simulink model "AMR_MoboticControlUnit_23b"  (R2023b)
settings: Solver=VariableStepAuto  StartTime=0.0  StopTime=10.0  RelTol=1e-3
values from neighbouring files (symbols this model uses):
  vehicle_track = 877    [param.mat]
  vehicle_wheelbase = 2367    [param.mat]
undefined symbols (not defined in the file or in its folder): boost_speed_multiplier, max_speed_multiplier
libraries: simulink_extras x3
settings Model: Creator=matlab.cut  LastModifiedBy=matlab.cut

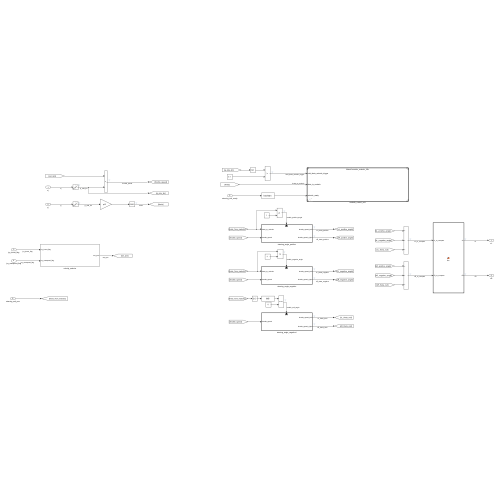
[thumbnail: Simulink's stored preview of the top-level diagram]
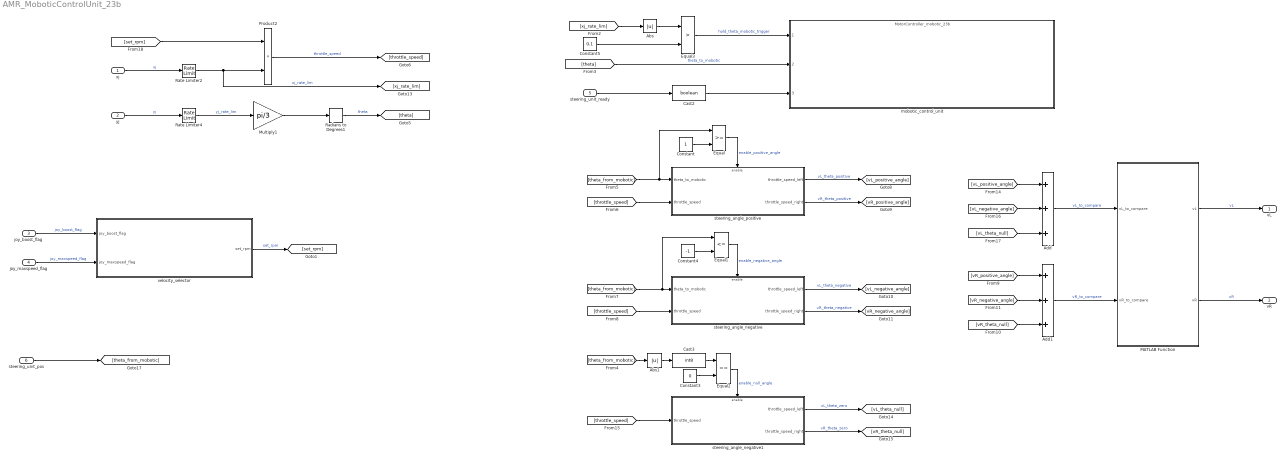
== system AMR_MoboticControlUnit_23b ==
  xj : Inport
  yj : Inport  Port=2
  joy_boost_flag : Inport  Port=3
  joy_maxspeed_flag : Inport  Port=4
  steering_unit_ready : Inport  Port=5
  steering_unit_pos : Inport  Port=6
  Abs : Abs  SaturateOnIntegerOverflow=off
  Abs1 : Abs  SaturateOnIntegerOverflow=off
  Add : Sum  Inputs=+++
  Add1 : Sum  Inputs=+++
  Cast2 : DataTypeConversion  OutDataTypeStr=boolean  SaturateOnIntegerOverflow=off  RndMeth=Floor
  Cast3 : DataTypeConversion  OutDataTypeStr=int8  SaturateOnIntegerOverflow=off  RndMeth=Floor
  Constant : Constant
  Constant3 : Constant  Value=0
  Constant4 : Constant  Value=-1
  Constant5 : Constant  Value=0.1
  Equal : RelationalOperator  OutDataTypeStr=boolean  RndMeth=Simplest  InputSameDT=off
  Equal1 : RelationalOperator  Operator=<=  OutDataTypeStr=boolean  RndMeth=Simplest  InputSameDT=off
  Equal2 : RelationalOperator  Operator===  OutDataTypeStr=boolean  RndMeth=Simplest  InputSameDT=off
  Equal3 : RelationalOperator  Operator=>  OutDataTypeStr=boolean  RndMeth=Simplest  InputSameDT=off
  MATLAB Function : MATLAB Function  TreatAsAtomicUnit=on
  Multiply1 : Gain  Gain=pi/3
  Product2 : Product
  Radians to Degrees1 : simulink_extras/Transformations/Radians to Degrees
  Rate Limiter2 : RateLimiter  SampleTimeMode=inherited
  Rate Limiter4 : RateLimiter  RisingSlewLimit=0.8  FallingSlewLimit=-0.8  SampleTimeMode=inherited
  mobotic_control_unit : ModelReference  ModelNameDialog=MotorController_mobotic_23b.slx  SimulationMode=Normal  ModelReferenceVersion=1.44
  steering_angle_negative : Subsystem
  steering_angle_negative1 : Subsystem
  steering_angle_positive : Subsystem
  velocity_selector : Subsystem
  vL : Outport
  vR : Outport  Port=2
  wires:
  [theta_from_mobotic] -> Abs1/1
  Abs1/1 -> Cast3/1
  steering_unit_ready/1 -> Cast2/1
  yj/1 -> Rate Limiter4/1  "yj"
  Cast2/1 -> mobotic_control_unit/3
  Rate Limiter2/1 -> [xj_rate_lim], Product2/2  "xj_rate_lim"
  [throttle_speed] -> steering_angle_negative1/1(throttle_speed)
  Abs/1 -> Equal3/1
  MATLAB Function/1(vL) -> vL/1  "vL"
  Add1/1 -> MATLAB Function/2(vR_to_compare)  "vR_to_compare"
  Constant4/1 -> Equal1/2
  Equal/1 -> steering_angle_positive/Enable  "enable_positive_angle"
  [vL_theta_null] -> Add/3
  steering_unit_pos/1 -> [theta_from_mobotic]
  [theta_from_mobotic] -> Equal/1, steering_angle_positive/1(theta_to_mobotic)
  Product2/1 -> [throttle_speed]  "throttle_speed"
  Constant3/1 -> Equal2/2
  [set_rpm] -> Product2/1
  [vL_negative_angle] -> Add/2
  Equal3/1 -> mobotic_control_unit/1  "hold_theta_mobotic_trigger"
  [vR_theta_null] -> Add1/3
  Cast3/1 -> Equal2/1
  [vR_negative_angle] -> Add1/2
  MATLAB Function/2(vR) -> vR/1  "vR"
  Rate Limiter4/1 -> Multiply1/1  "yj_rate_lim"
  steering_angle_negative/1(throttle_speed_left) -> [vL_negative_angle]  "vL_theta_negative"
  Constant/1 -> Equal/2
  xj/1 -> Rate Limiter2/1  "xj"
  [vR_positive_angle] -> Add1/1
  Constant5/1 -> Equal3/2
  steering_angle_positive/2(throttle_speed_right) -> [vR_positive_angle]  "vR_theta_positive"
  [xj_rate_lim] -> Abs/1
  [theta_from_mobotic] -> steering_angle_negative/1(theta_to_mobotic), Equal1/1
  steering_angle_negative/2(throttle_speed_right) -> [vR_negative_angle]  "vR_theta_negative"
  Radians to Degrees1/1 -> [theta]  "theta"
  Add/1 -> MATLAB Function/1(vL_to_compare)  "vL_to_compare"
  Equal2/1 -> steering_angle_negative1/Enable  "enable_null_angle"
  [vL_positive_angle] -> Add/1
  steering_angle_negative1/1(throttle_speed_left) -> [vL_theta_null]  "vL_theta_zero"
  [theta] -> mobotic_control_unit/2  "theta_to_mobotic"
  [throttle_speed] -> steering_angle_negative/2(throttle_speed)
  Multiply1/1 -> Radians to Degrees1/1
  steering_angle_positive/1(throttle_speed_left) -> [vL_positive_angle]  "vL_theta_positive"
  Equal1/1 -> steering_angle_negative/Enable  "enable_negative_angle"
  steering_angle_negative1/2(throttle_speed_right) -> [vR_theta_null]  "vR_theta_zero"
  [throttle_speed] -> steering_angle_positive/2(throttle_speed)
  velocity_selector/1(set_rpm) -> [set_rpm]  "set_rpm"
  joy_boost_flag/1 -> velocity_selector/1(joy_boost_flag)  "joy_boost_flag"
  joy_maxspeed_flag/1 -> velocity_selector/2(joy_maxspeed_flag)  "joy_maxspeed_flag"

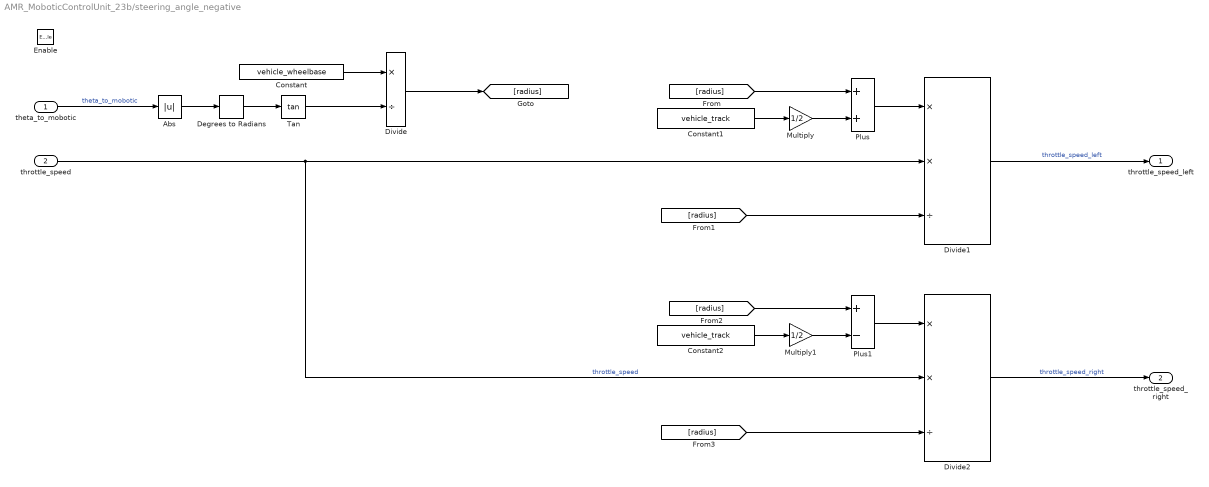
== system AMR_MoboticControlUnit_23b/steering_angle_negative ==
  theta_to_mobotic : Inport
  throttle_speed : Inport  Port=2
  Enable : EnablePort
  Abs : Abs  SaturateOnIntegerOverflow=off
  Constant : Constant  Value=vehicle_wheelbase
  Constant1 : Constant  Value=vehicle_track
  Constant2 : Constant  Value=vehicle_track
  Degrees to Radians : simulink_extras/Transformations/Degrees to Radians
  Divide : Product  Inputs=*/
  Divide1 : Product  Inputs=**/
  Divide2 : Product  Inputs=**/
  Multiply : Gain  Gain=1/2
  Multiply1 : Gain  Gain=1/2
  Plus : Sum
  Plus1 : Sum  Inputs=+-
  Tan : Trigonometry  Operator=tan
  throttle_speed_left : Outport  OutputWhenDisabled=reset  InitialOutput=[0]
  throttle_speed_right : Outport  Port=2  OutputWhenDisabled=reset  InitialOutput=[0]
  wires:
  Constant2/1 -> Multiply1/1
  Plus1/1 -> Divide2/1
  throttle_speed/1 -> Divide1/2, Divide2/2  "throttle_speed"
  Divide2/1 -> throttle_speed_right/1  "throttle_speed_right"
  [radius] -> Plus1/1
  Multiply1/1 -> Plus1/2
  [radius] -> Divide2/3
  [radius] -> Divide1/3
  Multiply/1 -> Plus/2
  [radius] -> Plus/1
  Divide1/1 -> throttle_speed_left/1  "throttle_speed_left"
  Plus/1 -> Divide1/1
  Constant1/1 -> Multiply/1
  Tan/1 -> Divide/2
  Divide/1 -> [radius]
  Constant/1 -> Divide/1
  Degrees to Radians/1 -> Tan/1
  Abs/1 -> Degrees to Radians/1
  theta_to_mobotic/1 -> Abs/1  "theta_to_mobotic"

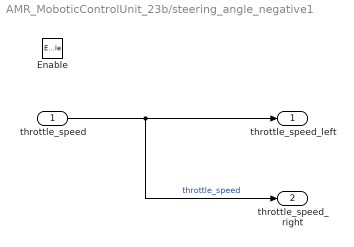
== system AMR_MoboticControlUnit_23b/steering_angle_negative1 ==
  throttle_speed : Inport
  Enable : EnablePort
  throttle_speed_left : Outport  OutputWhenDisabled=reset  InitialOutput=[0]
  throttle_speed_right : Outport  Port=2  OutputWhenDisabled=reset  InitialOutput=[0]
  wires:
  throttle_speed/1 -> throttle_speed_right/1, throttle_speed_left/1  "throttle_speed"

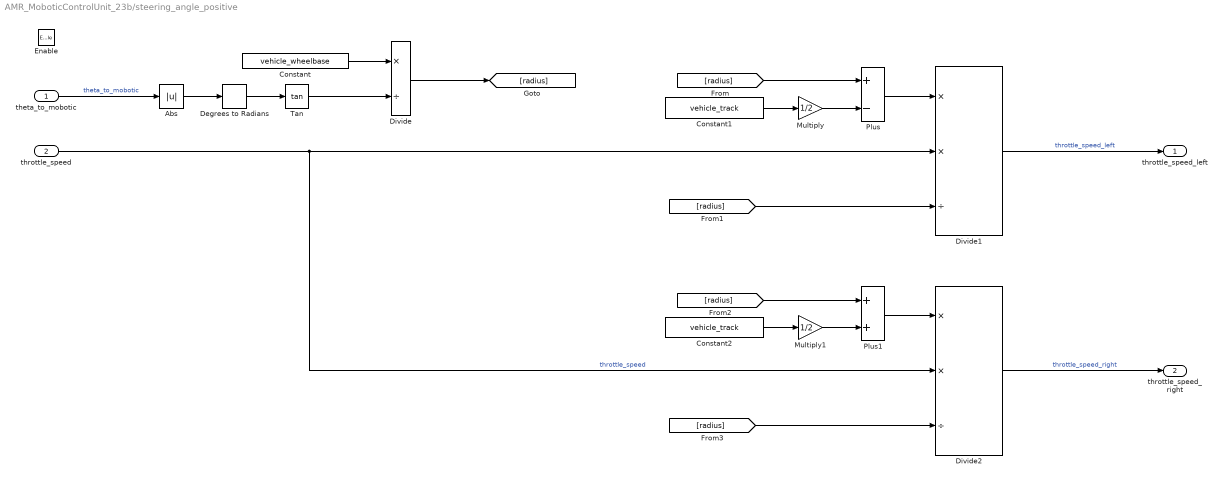
== system AMR_MoboticControlUnit_23b/steering_angle_positive ==
  theta_to_mobotic : Inport
  throttle_speed : Inport  Port=2
  Enable : EnablePort
  Abs : Abs  SaturateOnIntegerOverflow=off
  Constant : Constant  Value=vehicle_wheelbase
  Constant1 : Constant  Value=vehicle_track
  Constant2 : Constant  Value=vehicle_track
  Degrees to Radians : simulink_extras/Transformations/Degrees to Radians
  Divide : Product  Inputs=*/
  Divide1 : Product  Inputs=**/
  Divide2 : Product  Inputs=**/
  Multiply : Gain  Gain=1/2
  Multiply1 : Gain  Gain=1/2
  Plus : Sum  Inputs=+-
  Plus1 : Sum
  Tan : Trigonometry  Operator=tan
  throttle_speed_left : Outport  OutputWhenDisabled=reset  InitialOutput=[0]
  throttle_speed_right : Outport  Port=2  OutputWhenDisabled=reset  InitialOutput=[0]
  wires:
  theta_to_mobotic/1 -> Abs/1  "theta_to_mobotic"
  Abs/1 -> Degrees to Radians/1
  Degrees to Radians/1 -> Tan/1
  Constant/1 -> Divide/1
  Divide/1 -> [radius]
  Tan/1 -> Divide/2
  Constant1/1 -> Multiply/1
  Plus/1 -> Divide1/1
  Divide1/1 -> throttle_speed_left/1  "throttle_speed_left"
  [radius] -> Plus/1
  Multiply/1 -> Plus/2
  [radius] -> Divide1/3
  [radius] -> Divide2/3
  Multiply1/1 -> Plus1/2
  [radius] -> Plus1/1
  Divide2/1 -> throttle_speed_right/1  "throttle_speed_right"
  throttle_speed/1 -> Divide2/2, Divide1/2  "throttle_speed"
  Plus1/1 -> Divide2/1
  Constant2/1 -> Multiply1/1

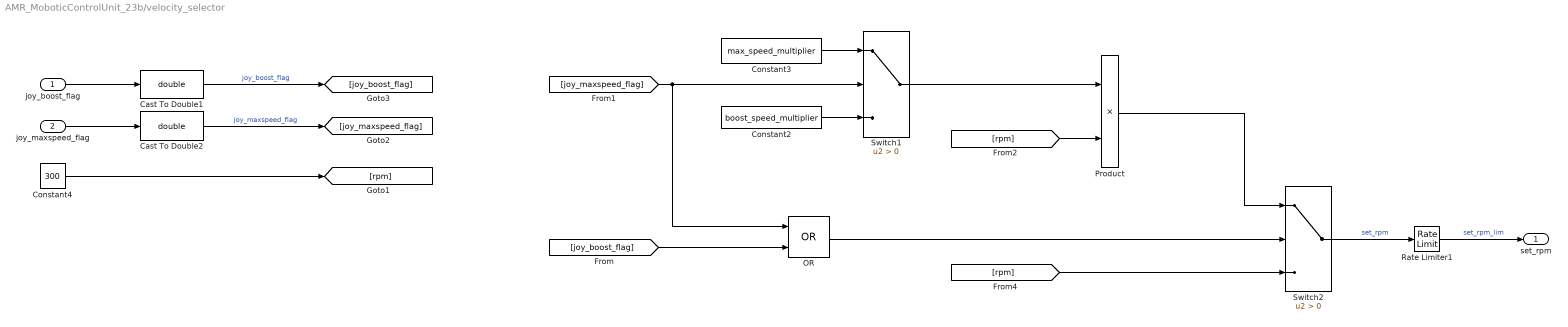
== system AMR_MoboticControlUnit_23b/velocity_selector ==
  joy_boost_flag : Inport
  joy_maxspeed_flag : Inport  Port=2
  Cast To Double1 : DataTypeConversion  OutDataTypeStr=double  SaturateOnIntegerOverflow=off  RndMeth=Floor
  Cast To Double2 : DataTypeConversion  OutDataTypeStr=double  SaturateOnIntegerOverflow=off  RndMeth=Floor
  Constant2 : Constant  Value=boost_speed_multiplier
  Constant3 : Constant  Value=max_speed_multiplier
  Constant4 : Constant  Value=300  VectorParams1D=off
  OR : Logic  Operator=OR  AllPortsSameDT=off  OutDataTypeStr=boolean
  Product : Product
  Rate Limiter1 : RateLimiter  RisingSlewLimit=800  FallingSlewLimit=-1400  SampleTimeMode=inherited
  Switch1 : Switch  Criteria=u2 > Threshold  SaturateOnIntegerOverflow=off  InputSameDT=off
  Switch2 : Switch  Criteria=u2 > Threshold  SaturateOnIntegerOverflow=off  InputSameDT=off
  set_rpm : Outport
  wires:
  Cast To Double2/1 -> [joy_maxspeed_flag]  "joy_maxspeed_flag"
  Cast To Double1/1 -> [joy_boost_flag]  "joy_boost_flag"
  joy_boost_flag/1 -> Cast To Double1/1
  joy_maxspeed_flag/1 -> Cast To Double2/1
  [joy_boost_flag] -> OR/2
  Switch2/1 -> Rate Limiter1/1  "set_rpm"
  [joy_maxspeed_flag] -> Switch1/2, OR/1
  Constant2/1 -> Switch1/3
  [rpm] -> Product/2
  Constant4/1 -> [rpm]
  Constant3/1 -> Switch1/1
  [rpm] -> Switch2/3
  OR/1 -> Switch2/2
  Switch1/1 -> Product/1
  Product/1 -> Switch2/1
  Rate Limiter1/1 -> set_rpm/1  "set_rpm_lim"

== matlab function AMR_MoboticControlUnit_23b/MATLAB Function ==
  data: vL_to_compare input; vL output; vR_to_compare input; vR output
function [vL, vR] = fcn(vL_to_compare, vR_to_compare)

max_curtis_speed = 3000; % rpm

if abs(vL_to_compare) >= max_curtis_speed
    vR = vR_to_compare * (max_curtis_speed / abs(vL_to_compare));
    vL = sign(vL_to_compare) * max_curtis_speed;
elseif abs(vR_to_compare) >= max_curtis_speed
    vL = vL_to_compare * (max_curtis_speed / abs(vR_to_compare));
    vR = sign(vR_to_compare) * max_curtis_speed;
else
    vL = vL_to_compare;
    vR = vR_to_compare;
end
